simulink model "lab2"  (R2016b)
settings: Solver=VariableStepAuto  StartTime=0.0  StopTime=50  RelTol=1e-3
libraries: simulink x1
settings Model: Creator=guilherme.mercurio  LastModifiedBy=guilherme.mercurio

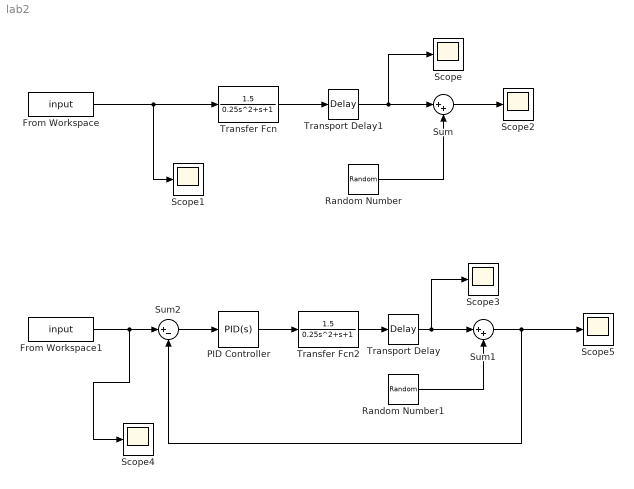
== system lab2 ==
  From Workspace : FromWorkspace  VariableName=input
  From Workspace1 : FromWorkspace  VariableName=input
  PID Controller : simulink/Continuous/PID Controller  Controller=PID  TimeDomain=Continuous-time  SampleTime=-1  IntegratorMethod=Forward Euler  FilterMethod=Forward Euler  Form=Parallel  UseFilter=on  ControllerParametersSource=internal  P=1  I=1  D=0  N=100  InitialConditionSource=internal  InitialConditionForIntegrator=0  InitialConditionForFilter=0  ExternalReset=none  LimitOutput=off  UpperSaturationLimit=inf  LowerSaturationLimit=-inf  LinearizeAsGain=on  AntiWindupMode=none  Kb=1  TrackingMode=off  Kt=1  PParamMin=[]  PParamMax=[]  IParamMin=[]  IParamMax=[]  DParamMin=[]  DParamMax=[]  NParamMin=[]  NParamMax=[]  KbParamMin=[]  KbParamMax=[]  KtParamMin=[]  KtParamMax=[]  POutMin=[]  POutMax=[]  IOutMin=[]  IOutMax=[]  DOutMin=[]  DOutMax=[]  NOutMin=[]  NOutMax=[]  KbOutMin=[]  KbOutMax=[]  KtOutMin=[]  KtOutMax=[]  IntegratorOutMin=[]  IntegratorOutMax=[]  FilterOutMin=[]  FilterOutMax=[]  SumOutMin=[]  SumOutMax=[]  SumI1OutMin=[]  SumI1OutMax=[]  SumI2OutMin=[]  SumI2OutMax=[]  SumI3OutMin=[]  SumI3OutMax=[]  SumDOutMin=[]  SumDOutMax=[]  SaturationOutMin=[]  SaturationOutMax=[]  IntegratorContinuousStateAttributes=''  IntegratorStateMustResolveToSignalObject=off  IntegratorRTWStateStorageClass=Auto  FilterContinuousStateAttributes=''  FilterStateMustResolveToSignalObject=off  FilterRTWStateStorageClass=Auto  DifferentiatorICPrevScaledInput=0  DifferentiatorOutMin=[]  DifferentiatorOutMax=[]
  Random Number : RandomNumber  Variance=0.01  SampleTime=0.1
  Random Number1 : RandomNumber  Variance=0.01  SampleTime=0.1
  Scope{,1..5} (6 alike) : Scope
  Sum : Sum  Inputs=|++
  Sum1 : Sum  Inputs=|++
  Sum2 : Sum  Inputs=|+-
  Transfer Fcn : TransferFcn  Numerator=[1.5]  Denominator=[0.25 1 1]
  Transfer Fcn2 : TransferFcn  Numerator=[1.5]  Denominator=[0.25 1 1]
  Transport Delay : TransportDelay
  Transport Delay1 : TransportDelay  DelayTime=1.25
  wires:
  Random Number/1 -> Sum/2
  Sum/1 -> Scope2/1
  From Workspace/1 -> Scope1/1, Transfer Fcn/1
  Transfer Fcn/1 -> Transport Delay1/1
  Random Number1/1 -> Sum1/2
  Sum1/1 -> Sum2/2, Scope5/1
  From Workspace1/1 -> Sum2/1, Scope4/1
  Transfer Fcn2/1 -> Transport Delay/1
  Transport Delay/1 -> Scope3/1, Sum1/1
  PID Controller/1 -> Transfer Fcn2/1
  Sum2/1 -> PID Controller/1
  Transport Delay1/1 -> Scope/1, Sum/1
